simulink model "lab2_2017"  (R2017b)
settings: Solver=VariableStepAuto  StartTime=0.0  StopTime=500  RelTol=1e-4
settings Model: Creator=razrab-ytka  LastModifiedBy=razrab-ytka
settings DataIOCC: ReturnWorkspaceOutputs=on
settings DebuggingCC: UnconnectedInputMsg=none  UnconnectedOutputMsg=none  UnconnectedLineMsg=none
settings ModelReferenceCC: EnableRefExpFcnMdlSchedulingChecks=off
settings SFSimCC: SimUseLocalCustomCode=on
settings RTWCC: Description=Generic Real-Time Target  RTWUseLocalCustomCode=on

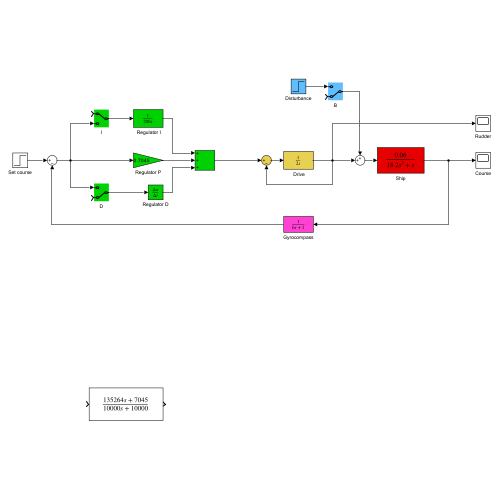
[thumbnail: Simulink's stored preview of the top-level diagram]
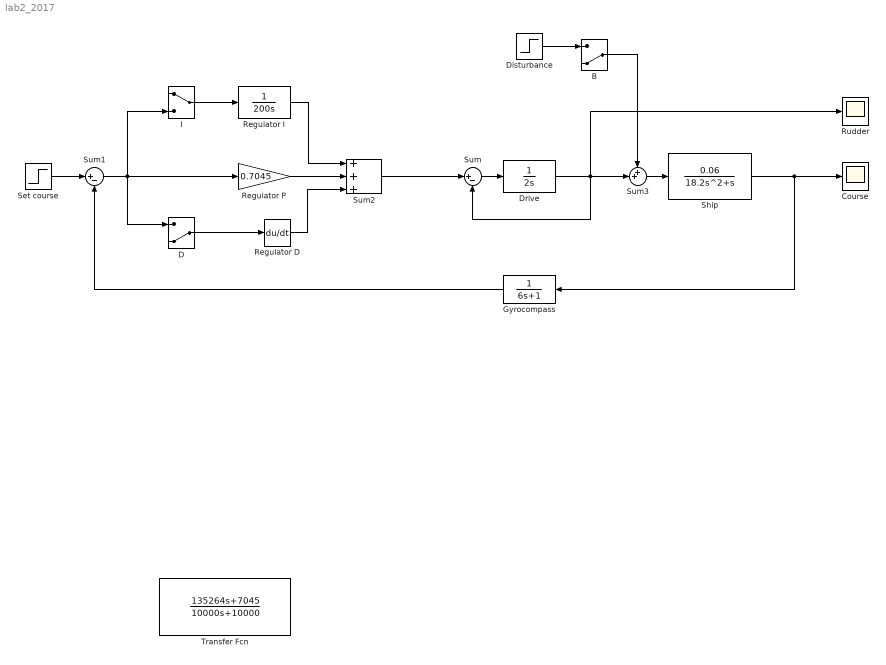
== system lab2_2017 ==
  " Drive" : TransferFcn  Denominator=[2 0]
  " Regulator I" : TransferFcn  Denominator=[200 0]
  B : ManualSwitch  CurrentSetting=0
  Course : Scope
  D : ManualSwitch  CurrentSetting=0
  Disturbance : Step  SampleTime=0
  Gyrocompass : TransferFcn  Denominator=[6 1]
  I : ManualSwitch
  Regulator D : Derivative
  Regulator P : Gain  Gain=0.7045
  Rudder : Scope
  Set course : Step  Time=0  After=10  SampleTime=0
  Ship : TransferFcn  Numerator=[0.06]  Denominator=[18.2 1 0]
  Sum : Sum  Inputs=|+-
  Sum1 : Sum  Inputs=|+-
  Sum2 : Sum  Inputs=+++
  Sum3 : Sum  Inputs=++|
  Transfer Fcn : TransferFcn  Numerator=[135264 7045]  Denominator=[10000 10000]
  wires:
  Sum/1 -> " Drive"/1
  Ship/1 -> Gyrocompass/1, Course/1
  Gyrocompass/1 -> Sum1/2
  " Regulator I"/1 -> Sum2/1
  Sum2/1 -> Sum/1
  Sum1/1 -> I/2, D/1, Regulator P/1
  Set course/1 -> Sum1/1
  I/1 -> " Regulator I"/1
  Sum3/1 -> Ship/1
  B/1 -> Sum3/1
  Disturbance/1 -> B/1
  " Drive"/1 -> Sum3/2, Sum/2, Rudder/1
  Regulator D/1 -> Sum2/3
  Regulator P/1 -> Sum2/2
  D/1 -> Regulator D/1
